simulink model "Lab_1_53"  (R2025b)
settings: Solver=ode4  StartTime=0.0  StopTime=10.0  FixedStep=0.2  RelTol=1e-3
settings Model: Creator=james  LastModifiedBy=james
settings DataIOCC: ReturnWorkspaceOutputs=off

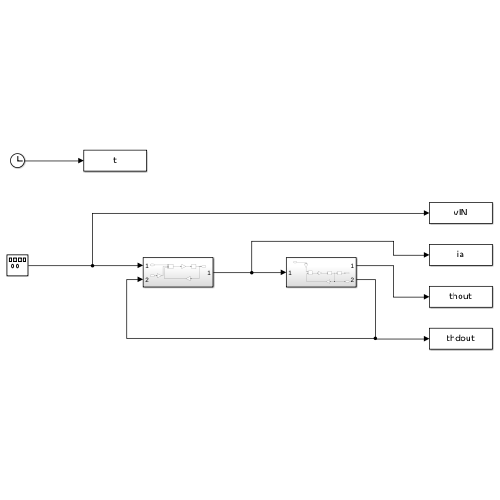
[thumbnail: Simulink's stored preview of the top-level diagram]
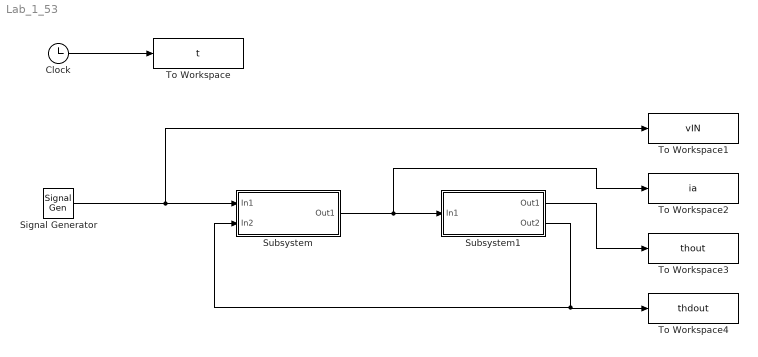
== system Lab_1_53 ==
  Clock : Clock
  Signal Generator : SignalGenerator  Units=rad/sec
  Subsystem : Subsystem
  Subsystem1 : Subsystem
  To Workspace : ToWorkspace  VariableName=t  SaveFormat=Timeseries  SampleTime=-1
  To Workspace1 : ToWorkspace  VariableName=vIN  SaveFormat=Timeseries  SampleTime=-1
  To Workspace2 : ToWorkspace  VariableName=ia  SaveFormat=Timeseries  SampleTime=-1
  To Workspace3 : ToWorkspace  VariableName=thout  SaveFormat=Timeseries  SampleTime=-1
  To Workspace4 : ToWorkspace  VariableName=thdout  SaveFormat=Timeseries  SampleTime=-1
  wires:
  Clock/1 -> To Workspace/1
  Signal Generator/1 -> To Workspace1/1, Subsystem/1(In1)
  Subsystem/1(Out1) -> To Workspace2/1, Subsystem1/1(In1)
  Subsystem1/1(Out1) -> To Workspace3/1
  Subsystem1/2(Out2) -> Subsystem/2(In2), To Workspace4/1

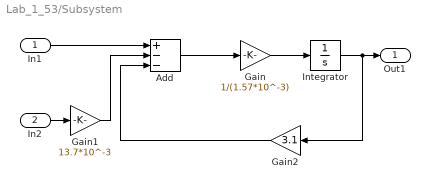
== system Lab_1_53/Subsystem ==
  In1 : Inport
  In2 : Inport  Port=2
  Add : Sum  Inputs=+--
  Gain : Gain  Gain=1/(1.57*10^-3)
  Gain1 : Gain  Gain=13.7*10^-3
  Gain2 : Gain  Gain=3.1
  Integrator : Integrator
  Out1 : Outport
  wires:
  Integrator/1 -> Gain2/1, Out1/1
  Gain/1 -> Integrator/1
  Add/1 -> Gain/1
  In1/1 -> Add/1
  In2/1 -> Gain1/1
  Gain1/1 -> Add/2
  Gain2/1 -> Add/3

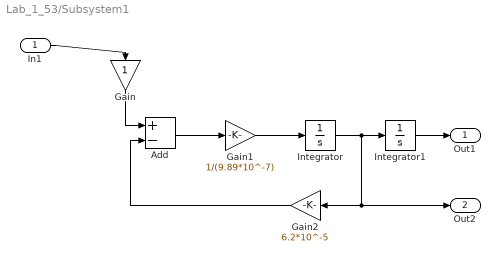
== system Lab_1_53/Subsystem1 ==
  In1 : Inport
  Add : Sum  Inputs=+-
  Gain : Gain
  Gain1 : Gain  Gain=1/(9.89*10^-7)
  Gain2 : Gain  Gain=6.2*10^-5
  Integrator : Integrator
  Integrator1 : Integrator
  Out1 : Outport
  Out2 : Outport  Port=2
  wires:
  In1/1 -> Gain/1
  Gain/1 -> Add/1
  Add/1 -> Gain1/1
  Gain1/1 -> Integrator/1
  Integrator/1 -> Out2/1, Gain2/1, Integrator1/1
  Integrator1/1 -> Out1/1
  Gain2/1 -> Add/2
